simulink model "EX4_ex6"  (R2018b)
settings: Solver=VariableStepAuto  StartTime=0.0  StopTime=10.0  RelTol=1e-3
settings Model: Creator=吳俊逸  LastModifiedBy=吳俊逸

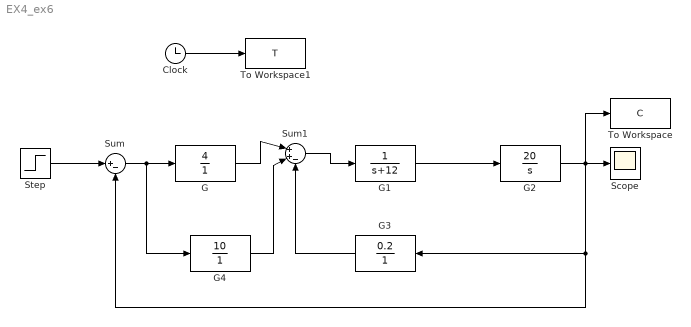
== system EX4_ex6 ==
  Clock : Clock
  G : TransferFcn  Numerator=[4]  Denominator=[1]
  G1 : TransferFcn  Denominator=[1 12]
  G2 : TransferFcn  Numerator=[20]  Denominator=[1 0]
  G3 : TransferFcn  Numerator=[0.2]  Denominator=[1]
  G4 : TransferFcn  Numerator=[10]  Denominator=[1 ]
  Scope : Scope
  Step : Step  Time=0  SampleTime=0
  Sum : Sum  Inputs=|+-
  Sum1 : Sum  Inputs=|++-
  To Workspace : ToWorkspace  VariableName=C  SampleTime=-1
  To Workspace1 : ToWorkspace  VariableName=T  SampleTime=-1
  wires:
  Step/1 -> Sum/1
  Sum/1 -> G4/1, G/1
  G/1 -> Sum1/1
  G4/1 -> Sum1/2
  G3/1 -> Sum1/3
  Sum1/1 -> G1/1
  G1/1 -> G2/1
  G2/1 -> To Workspace/1, Scope/1, Sum/2, G3/1
  Clock/1 -> To Workspace1/1
